simulink model "HalfCar_F"  (R2022a)
settings: Solver=VariableStepAuto  StartTime=0.0  StopTime=10.0  RelTol=1e-3
PreLoadFcn:
  | Lf = 0.9;    % front hub displacement from body gravity center (m)
  | Lr = 1.2;    % rear hub displacement from body gravity center (m)
  | m = 1200;   % body mass (kg)
  | I = 2100;  % body moment of inertia about y-axis in (kg m^2)
  | Kf = 28000;  % front suspension stiffness in (N/m)
  | Kr = 21000;  % rear suspension stiffness in (N/m)
  | Cf = 2500;   % front suspension damping in (N sec/m)
  | Cr = 2000;   % rear suspension damping in (N sec/m)
settings Model: Creator=SK  LastModifiedBy=SK

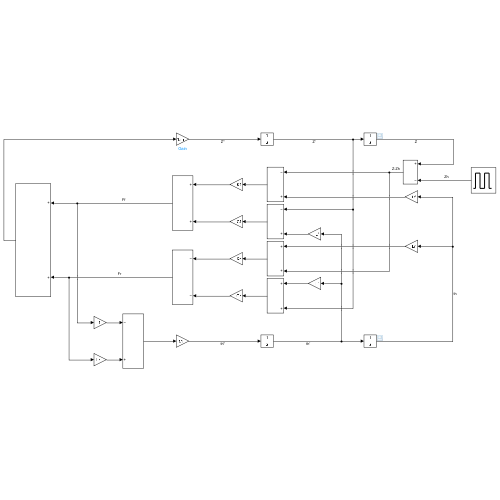
[thumbnail: Simulink's stored preview of the top-level diagram]
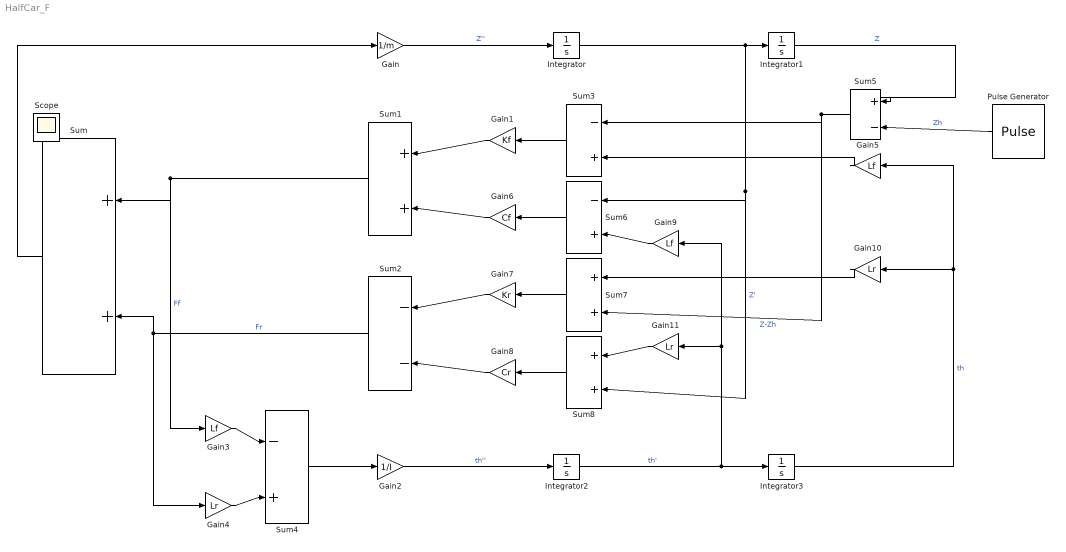
== system HalfCar_F ==
  Gain : Gain  Gain=1/m
  Gain1 : Gain  Gain=Kf
  Gain10 : Gain  Gain=Lr
  Gain11 : Gain  Gain=Lr
  Gain2 : Gain  Gain=1/I
  Gain3 : Gain  Gain=Lf
  Gain4 : Gain  Gain=Lr
  Gain5 : Gain  Gain=Lf
  Gain6 : Gain  Gain=Cf
  Gain7 : Gain  Gain=Kr
  Gain8 : Gain  Gain=Cr
  Gain9 : Gain  Gain=Lf
  Integrator{,1..3} (4 alike) : Integrator
  Pulse Generator : DiscretePulseGenerator  PulseType=Time based  Period=10  PulseWidth=10  PhaseDelay=2
  Sum{,1,7..8} (4 alike) : Sum  Inputs=+|+
  Sum2 : Sum  Inputs=-|-
  Sum3 : Sum  Inputs=-|+
  Sum4 : Sum  Inputs=-|+
  Sum5 : Sum  Inputs=+|-
  Sum6 : Sum  Inputs=-|+
  Scope : Scope
  wires:
  Integrator/1 -> Sum8/2, Sum6/1, Integrator1/1  "Z'"
  Integrator1/1 -> Sum5/1  "Z"
  Gain/1 -> Integrator/1  "Z''"
  Sum/1 -> Gain/1
  Sum1/1 -> Gain3/1, Sum/1  "Ff"
  Sum2/1 -> Sum/2, Gain4/1  "Fr"
  Pulse Generator/1 -> Sum5/2  "Zh"
  Gain1/1 -> Sum1/1
  Sum3/1 -> Gain1/1
  Gain2/1 -> Integrator2/1  "th''"
  Integrator3/1 -> Gain10/1, Gain5/1  "th"
  Integrator2/1 -> Gain11/1, Gain9/1, Integrator3/1  "th'"
  Sum4/1 -> Gain2/1
  Gain3/1 -> Sum4/1
  Gain4/1 -> Sum4/2
  Gain5/1 -> Sum3/2
  Sum5/1 -> Sum7/2, Sum3/1  "Z-Zh"
  Gain6/1 -> Sum1/2
  Sum6/1 -> Gain6/1
  Gain8/1 -> Sum2/2
  Sum8/1 -> Gain8/1
  Gain7/1 -> Sum2/1
  Sum7/1 -> Gain7/1
  Gain9/1 -> Sum6/2
  Gain10/1 -> Sum7/1
  Gain11/1 -> Sum8/1
